simulink model "Spunto4"  (R2022a)
settings: Solver=VariableStepAuto  StartTime=0.0  StopTime=15  RelTol=1e-3
settings Model: Creator=bryan  LastModifiedBy=bryan

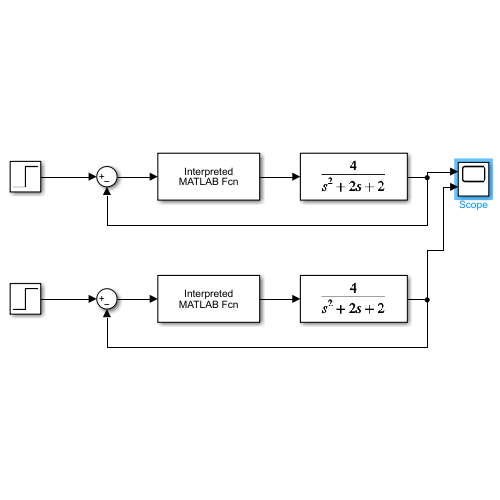
[thumbnail: Simulink's stored preview of the top-level diagram]
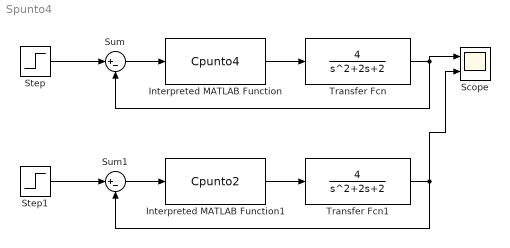
== system Spunto4 ==
  Interpreted MATLAB Function : MATLABFcn  MATLABFcn=Cpunto4
  Interpreted MATLAB Function1 : MATLABFcn  MATLABFcn=Cpunto2
  Scope : Scope  NumInputPorts=2
  Step : Step  SampleTime=0
  Step1 : Step  SampleTime=0
  Sum : Sum  Inputs=|+-
  Sum1 : Sum  Inputs=|+-
  Transfer Fcn : TransferFcn  Numerator=[4]  Denominator=[1 2 2]
  Transfer Fcn1 : TransferFcn  Numerator=[4]  Denominator=[1 2 2]
  wires:
  Step/1 -> Sum/1
  Sum/1 -> Interpreted MATLAB Function/1
  Interpreted MATLAB Function/1 -> Transfer Fcn/1
  Transfer Fcn/1 -> Scope/1, Sum/2
  Interpreted MATLAB Function1/1 -> Transfer Fcn1/1
  Step1/1 -> Sum1/1
  Sum1/1 -> Interpreted MATLAB Function1/1
  Transfer Fcn1/1 -> Scope/2, Sum1/2
